simulink subsystem "SubSystemDrive"  (R2020b)
settings: Solver=VariableStepAuto  StartTime=0.0  StopTime=10.0  RelTol=1e-3
settings Model: Creator=kaebi  LastModifiedBy=kaebi

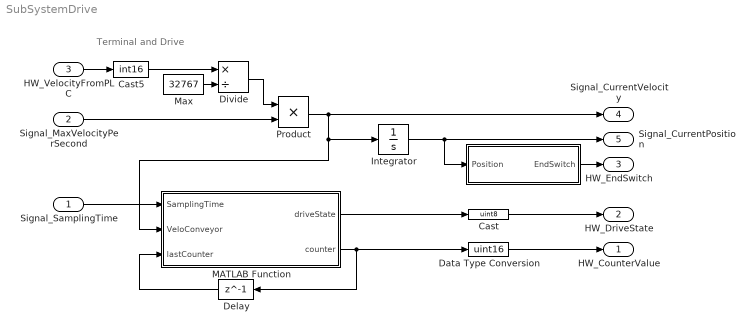
== system SubSystemDrive ==
  note: Terminal and Drive
  Signal_SamplingTime : Inport
  Signal_MaxVelocityPerSecond : Inport  Port=2
  HW_VelocityFromPLC : Inport  Port=3
  " " : MATLAB Function  TreatAsAtomicUnit=on
  Cast : DataTypeConversion  OutDataTypeStr=uint8
  Cast5 : DataTypeConversion  OutDataTypeStr=int16
  Data Type Conversion : DataTypeConversion  OutDataTypeStr=uint16  SaturateOnIntegerOverflow=on
  Delay : Delay  DelayLength=1
  Divide : Product  Inputs=*/
  Integrator : Integrator  InitialCondition=10  LimitOutput=on  LowerSaturationLimit=-1
  MATLAB Function : MATLAB Function  TreatAsAtomicUnit=on
  Max : Constant  Value=32767
  Product : Product
  HW_CounterValue : Outport
  HW_DriveState : Outport  Port=2
  HW_EndSwitch : Outport  Port=3  OutDataTypeStr=boolean
  Signal_CurrentVelocity : Outport  Port=4
  Signal_CurrentPosition : Outport  Port=5
  wires:
  Signal_MaxVelocityPerSecond/1 -> Product/2
  Signal_SamplingTime/1 -> MATLAB Function/1(SamplingTime)
  Cast5/1 -> Divide/1
  MATLAB Function/2(counter) -> Delay/1, Data Type Conversion/1
  Max/1 -> Divide/2
  Product/1 -> Signal_CurrentVelocity/1, Integrator/1, MATLAB Function/2(VeloConveyor)
  Data Type Conversion/1 -> HW_CounterValue/1
  MATLAB Function/1(driveState) -> Cast/1
  HW_VelocityFromPLC/1 -> Cast5/1
  Divide/1 -> Product/1
  Cast/1 -> HW_DriveState/1
  Delay/1 -> MATLAB Function/3(lastCounter)
  Integrator/1 -> " "/1(Position), Signal_CurrentPosition/1
  " "/1(EndSwitch) -> HW_EndSwitch/1

== matlab function SubSystemDrive/  ==
  data: Position input; EndSwitch output
function EndSwitch = EndSwitch(Position)

EndSwitch = true;
if (Position <= 0)
    EndSwitch = false;
end

== matlab function SubSystemDrive/MATLAB Function ==
  data: driveState output; SamplingTime input; VeloConveyor input; counter output; lastCounter input
function [driveState,counter] = GenericDriveTerminal(SamplingTime, VeloConveyor, lastCounter)
%%
%    VeloConveyor in Unit/s
%    SamplingTime in s
%    lastCounter 1count = 0.0001 Unit

%%
driveState = uint8(0);
driveState = bitset(driveState,1,1);    % Ready to enable
driveState = bitset(driveState,2,1);    % Ready 
if (VeloConveyor > 0)
    driveState = bitset(driveState,5,1);    % Moving Positive
elseif (VeloConveyor < 0)
    driveState = bitset(driveState,6,1);    % Moving Negative
end

diff = VeloConveyor*SamplingTime*10000;
counter = lastCounter+diff;
if (counter >= 65535)
    counter = mod(counter,65535);
elseif (counter < 0)
    counter = 65535 + counter;
end

end
